simulink model "vrtkoff_trace"  (Simulink 7.4)
settings: Solver=ode45  StartTime=0.0  StopTime=15  RelTol=1e-3
libraries: vrlib x3, aerospace x1
Description:
  | Plane Take-Off with Trajectory Tracing
  | 
  | This model is a variant of the vrtkoff example that shows how to trace trajectory of
  | a moving object (the plane) in the scene.
  | 
  | VR Tracer block adds the following behavior to the scene visualization:
  | 
  | A marker is placed at the current position of the traced object in regular time intervals
  | specified by the block sample time. Markers form a visible trace of the object's trajectory.
  | The distance between markers indicates the speed of the object at given position.
  | In addition, marker color can be dynamically set using the second block input to represent
  | another model property or status.
  | 
  | VR Tracer block allows you to specify the following parameters:
  | - Associated VRML File
  | - Parent node of markers to create  (useful when the traced object is inside other object in the scene hierarchy)
  | - General marker shape to be selected from the listbox (select None for displaying line / triads below only)
  | - Checkboxes to select whether you want to display trajectory as a line and/or axis-aligned triads
  | - Marker scale
  | - Marker color, to be defined in block input or in the block mask.
  | - Sample time
  | - Checkbox to ensure that a viewer window is open during simulation
  | 
  | In this example, a tetrahedron shape is used as a general shape marker, together with both trajectory line and triads.
settings Model: Creator=Straka  LastModifiedBy=Houska  CovMetricSettings=d  ExtModeTrigMode=oneshot  ExtModeArmWhenConnect=off
settings SolverCC: InsertRTBMode=Auto
settings DataIOCC: SaveOutput=off  SaveTime=off  SignalLoggingName=logsOut
settings OptimizationCC: BlockReduction=off  BooleanDataType=off  InlineInvariantSignals=on  InitFltsAndDblsToZero=on  EfficientMapNaN2IntZero=off
settings DebuggingCC: CheckExecutionContextPreStartOutputMsg=on  CheckExecutionContextRuntimeOutputMsg=on  SignalResolutionControl=TryResolveAllWithWarning  SolverPrmCheckMsg=none  MultiTaskDSMMsg=warning  MultiTaskCondExecSysMsg=none  StrictBusMsg=None
settings HardwareCC: TargetUnknown=on
settings ModelReferenceCC: UpdateModelReferenceTargets=IfOutOfDate
settings SFSimCC: SimGenerateEmlReport=off
settings RTWCC: IncludeERTFirstTime=on
settings GRTTargetCC: TargetFcnLib=ansi_tfl_tmw.mat

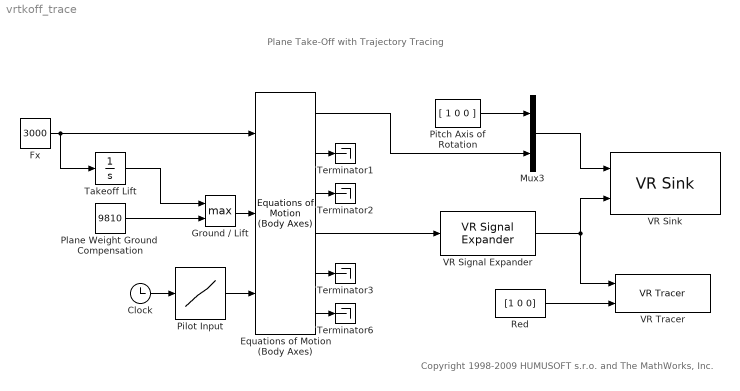
== system vrtkoff_trace ==
  note: Copyright 1998-2009 HUMUSOFT s.r.o. and The MathWorks, Inc.
  note: Plane Take-Off with Trajectory Tracing
  " Equations of Motion (Body Axes)" : aerospace/3DoF Equations of Motion / Equations of Motion (Body Axes)  SystemSampleTime=-1  v_ini=0  theta_ini=0  alpha_ini=0  q_ini=0  pos_ini=[0 0]  mass=1000  Iyy=1000  g=-9.81
  Clock : Clock
      settings: Decimation=10
  Fx : Constant  Value=3000  OutDataType=sfix(16)  OutScaling=2^0
  Ground / Lift : MinMax  Function=max  Inputs=2  OutDataType=sfix(16)  OutScaling=2^0  ZeroCross=off  SaturateOnIntegerOverflow=on  InputSameDT=on
  Mux3 : Mux  Inputs=2
  Pilot Input : Lookup  InputValues=[0 1 2 8 9 15]  Table=[0 0 -20 20 0 0]  OutDataType=sfix(16)  OutScaling=2^0  SaturateOnIntegerOverflow=on
  Pitch Axis of Rotation : Constant  Value=[ 1 0 0 ]  OutDataType=sfix(16)  OutScaling=2^0
  Plane Weight Ground  Compensation : Constant  Value=9810  OutDataType=sfix(16)  OutScaling=2^0
  Red : Constant  Value=[1 0 0]  OutDataType=sfix(16)  OutScaling=2^0
  Takeoff Lift : Integrator  LimitOutput=on  UpperSaturationLimit=11000  LowerSaturationLimit=-Inf  ZeroCross=off
  Terminator{1..3,6} (4 alike) : Terminator
  VR Signal Expander : vrlib/VR Signal Expander  SystemSampleTime=-1  outwidth=3  outidx=[3 2]
  VR Sink : vrlib/VR Sink  InstantiateOnLoad=on  SampleTime=0.05  ViewEnable=on  RemoteChange=off  RemoteView=off  FieldsWritten=Plane.rotation.4.1.double#Plane.translation.3.1.double  WorldFileName=vrtkoff.wrl  WorldDescription=VR Plane Take-Off  AutoView=on  VideoDimensions=[]  FigureProperties="{'Position', 'Name', 'Viewpoint', 'CameraBound', 'CameraDirection', 'CameraPosition', 'CameraUpVector', 'ZoomFactor', 'Antialiasing', 'Headlight', 'Lighting', 'NavPanel', 'StatusBar', 'ToolBar', 'Textures', 'Transparency', 'Wireframe', 'NavZones', 'NavMode', 'NavSpeed', 'Record2DCompressMethod', 'Record2DCompressQuality', 'Record2D', 'Record2DFileName', 'Record2DFPS'; [2.6000000000000000e+001  7.9000000000000000e+001  5.7600000000000000e+002  3.8000000000000000e+002], 'VR Plane Take-Off', 'Airport', 'on', [0.0000000000000000e+000  0.0000000000000000e+000 -1.0000000000000000e+000], [0.0000000000000000e+000  0.0000000000000000e+000  0.0000000000000000e+000], [0.0000000000000000e+000  1.0000000000000000e+000  0.0000000000000000e+000], [1.0000000000000000e+000], 'off', 'on', 'on', 'halfbar', 'off', 'on', 'on', 'on', 'off', 'off', 'fly', 'normal', 'auto', [7.5000000000000000e+001], 'off', '%f_anim_%n.avi', [1.5000000000000000e+001]}"
  VR Tracer : vrlib/VR Tracer  VrmlFile=vrtkoff.wrl  MarkerName=Tetrahedron  UseLines=on  UseTriads=on  MarkerScale=[1 1 1]  MarkerColorSelection=Block input  MarkerColor=red  rgbval=[1 0 0]  Ts=0.5  ForceViewerOpen=off
  wires:
  Pitch Axis of Rotation/1 -> Mux3/1
  VR Signal Expander/1 -> VR Sink/2, VR Tracer/1
  " Equations of Motion (Body Axes)"/2 -> Terminator1/1
  " Equations of Motion (Body Axes)"/3 -> Terminator2/1
  Ground / Lift/1 -> " Equations of Motion (Body Axes)"/2
  Takeoff Lift/1 -> Ground / Lift/1
  Plane Weight Ground  Compensation/1 -> Ground / Lift/2
  Clock/1 -> Pilot Input/1
  Pilot Input/1 -> " Equations of Motion (Body Axes)"/3
  Fx/1 -> " Equations of Motion (Body Axes)"/1, Takeoff Lift/1
  " Equations of Motion (Body Axes)"/6 -> Terminator6/1
  " Equations of Motion (Body Axes)"/5 -> Terminator3/1
  " Equations of Motion (Body Axes)"/1 -> Mux3/2
  " Equations of Motion (Body Axes)"/4 -> VR Signal Expander/1
  Red/1 -> VR Tracer/2
  Mux3/1 -> VR Sink/1
